simulink model "mbkKalman"  (R2018a)
settings: Solver=ode4  StartTime=0.0  StopTime=50  FixedStep=0.01  RelTol=1e-3
values from neighbouring files (symbols this model uses):
  A = [0 1;     -k/m -b/m]    [Kalman.m]    (also in fcn.m; temtProp.m = [0 1;-g/l 0]; untitled2.m)
  b = 5    [Kalman.m]    (also in fcn.m; untitled2.m)
  B = [0; 1/m]    [Kalman.m]    (also in fcn.m; temtProp.m = [0;1/(m*l^2)]; untitled2.m)
  C = [0 1]    [Kalman.m]    (also in fcn.m; temtProp.m = [1 0]; untitled2.m)
  k = 5    [Kalman.m]    (also in fcn.m; temtProp.m = 100; untitled2.m)
  m = 10    [Kalman.m]    (also in fcn.m; temtProp.m; untitled2.m)
undefined symbols (not defined in the file or in its folder): Continuous, Time
libraries: simulink x1, ctrlSharedLib x1
settings Model: Creator=Ali  LastModifiedBy=Ali

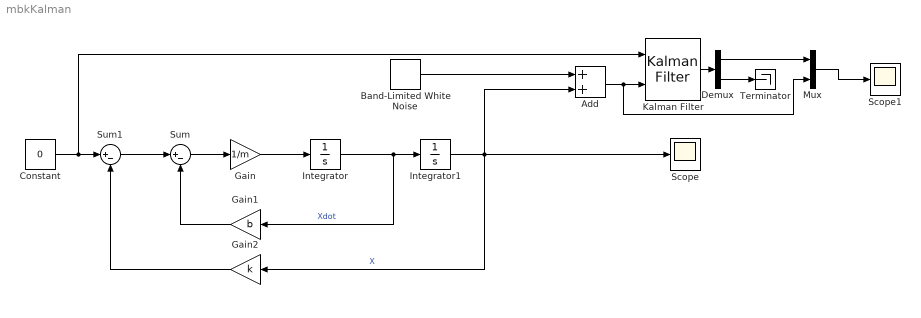
== system mbkKalman ==
  Add : Sum
  Band-Limited White Noise : simulink/Sources/Band-Limited White Noise  Cov=[0.1]  Ts=0.1  seed=[23341]
  Constant : Constant  Value=0
  Demux : Demux  Outputs=2
  Gain : Gain  Gain=1/m
  Gain1 : Gain  Gain=b
  Gain2 : Gain  Gain=k
  Integrator : Integrator
  Integrator1 : Integrator
  Kalman Filter : ctrlSharedLib/Kalman Filter  TimeDomain=Continuous-Time  UseCurrentEstimator=on  ModelSource=Individual A, B, C, D matrices  ModelSourceVariable=ss(0.95,1,1,0,1)  A=A  B=B  C=C  D=0  NumberOfStates=1  NumberOfInputs=1  NumberOfOutputs=1  InitialEstimateSource=Dialog  X0=[10 0]  P0=10  UseK=off  UseGH=off  NumberOfProcessNoiseInputs=1  G=1  TimeInvariantG=on  H=0  TimeInvariantH=on  Q=0.05  TimeInvariantQ=on  R=1  TimeInvariantR=on  N=0  TimeInvariantN=on  AddInputPort=on  AddEnablePort=off  OutputEstimatedY=off  OutputP=off  Ts=-1
      settings: SourceProductBaseCode=CT
  Mux : Mux  Inputs=2
  Scope : Scope
  Scope1 : Scope
  Sum : Sum  Inputs=|+-
  Sum1 : Sum  Inputs=|+-
  Terminator : Terminator
  wires:
  Integrator/1 -> Gain1/1, Integrator1/1  "Xdot"
  Integrator1/1 -> Add/2, Gain2/1, Scope/1  "X"
  Gain/1 -> Integrator/1
  Sum/1 -> Gain/1
  Gain1/1 -> Sum/2
  Sum1/1 -> Sum/1
  Gain2/1 -> Sum1/2
  Constant/1 -> Kalman Filter/1, Sum1/1
  Kalman Filter/1 -> Demux/1
  Demux/1 -> Mux/1
  Demux/2 -> Terminator/1
  Mux/1 -> Scope1/1
  Band-Limited White Noise/1 -> Add/1
  Add/1 -> Mux/2, Kalman Filter/2
